simulink model "usrp_4t12r_heatmap"  (R2018a)
settings: Solver=VariableStepDiscrete  StartTime=0.0  StopTime=inf  RelTol=1e-3
undefined symbols (not defined in the file): fft2, gather, get, gpuArray, parula, psBcoor, psWcen, rfcaptureC2Fsim, Time, tsRamp, us
libraries: neural x14, visionanalysis x8, dspobslib x8, dspfdesign x7, dspstat3 x5, dspbuff3 x2, visionsinks x2, commsdrhw_v2 x1, visiontextngfix x1, dspvision x1, visiontransforms x1, dspsigops x1
(part 1 of 4)
settings Model: SimulationMode=accelerator  Creator=Sky  LastModifiedBy=Sky
settings DataIOCC: SaveTime=off
settings OptimizationCC: DefaultUnderspecifiedDataType=single  EfficientMapNaN2IntZero=off  SimCompilerOptimization=on
settings DebuggingCC: ReadBeforeWriteMsg=DisableAll  WriteAfterWriteMsg=DisableAll  WriteAfterReadMsg=DisableAll  MultiTaskDSMMsg=none
settings HardwareCC: TargetBitPerPointer=64  TargetBitPerSizeT=64  TargetBitPerPtrDiffT=64  TargetLongLongMode=on  TargetIntDivRoundTo=Zero  TargetEndianess=LittleEndian  TargetWordSize=64  TargetHWDeviceType=MATLAB Host  ProdEqTarget=off
settings ModelReferenceCC: UpdateModelReferenceTargets=IfOutOfDate
settings SFSimCC: SFSimEcho=off
settings CodeAppCC: MaxIdLength=128  StateflowObjectComments=on
settings GRTTargetCC: TargetLangStandard=C89/C90 (ANSI)  CombineOutputUpdateFcns=off  GRTInterface=on

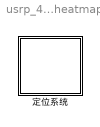
== system usrp_4t12r_heatmap ==
  定位系统 : Subsystem  mask{doSaveParam=on, mode=imaging mode, decimInterp=100, rxBits=logical(dec2bin(0:11)-48), txBits=logical(dec2bin(0:3)-48), rxCoor=single([linspace(-0.053*(12/2-0.5),0.053*(12/2-0.5),12)',zeros(12,2)]), txCoor=single([zeros(4,2),linspace(-0.138-0.053*3,-0.138,4)']), dCa=4.65+0.5, fRamp=2000, fCen=3.2e9, fBw=1e9, tPul=0.025e-3, trEdge=0, trThres=0, yLoDownFac=5, nCyclePF=4, lFftAng=64, lFftDis=128, tDelay=0.5, sFileBack='..\data\yLoCut_4t12r_background.mat', xMi=-3, xMa=3, yMi=1, yMa=4, zMi=-1.25, zMa=0.25, dxC=0.25, dyC=0.25, dzC=0.25, C2Fw=3, C2Fn=2, C2Fratio=0.5, lxW=1, lyW=1, lzW=1.5, tSam=3, nSam=3}
      mask prompts: doSaveParam "save parameters to workspace"; decimInterp "decimation factor"; rxBits "Rx bits"; txBits "Tx bits"; rxCoor "rx coordinates"; txCoor "tx coordinates"; dCa "cable length"; fRamp "ramp frequency"; fCen "center frequency"; fBw "bandwidth"; tPul "pulse width"; trEdge "triger edge"; trThres "triger threshold"; yLoDownFac "yLo downsample factor"; nCyclePF "cycles per frame (average time)"; lFftAng "angle FFT length"; lFftDis "dis FFT length"; tDelay "delay time"; sFileBack "background file path"; xMi "x min"; xMa "x max"; yMi "y min"; yMa "y max"; zMi "z min"; zMa "z max"; dxC "delta x coarse"; dyC "delta y coarse"; dzC "delta z coarse"; C2Fw "coarse to fine width"; C2Fn "coarse to fine cycle number"; C2Fratio "coarse to fine ratio"; lxW "window width x"; lyW "window width y"; lzW "window width z"; tSam "sample time"; nSam "sample number"
      mask init:
      | % Use get_param to obtain the selected string
      | mode = get_param(gcb,'mode');
      | 
      | if strcmp(mode,'get background mode') ...
      |         || strcmp(mode,'sample mode')
      |     evalin('base','clear');
      | end
      | 
      | % 天线和斜坡参数
      | nRx=size(rxBits,1);
      | nTx=size(txBits,1);
      | lFraw=100e6/decimInterp/fRamp*nRx*nTx*nCyclePF;
      | fSraw=100e6/decimInterp;
      | fSdown=fSraw/yLoDownFac;
      | fF=fSraw/lFraw;
      | lRampRaw=fSraw/fRamp;%length ramp raw
      | lRampDown=lRampRaw/yLoDownFac;%length ramp downsample
      | nPul=size(rxBits,2)+size(txBits,2)+1;
      | lPul=fSraw*tPul;%length pulse
      | 
      | dLambda=3e8/fCen;
      | fPm=fBw*fRamp/3e8;%frequency per meter
      | fD=fSdown/lFftDis;%frequency delta
      | fs=single(linspace(0,fSraw/yLoDownFac/2-fD,floor(lFftDis/2)));
      | ds=fs/fPm;
      | 
      | angMax=asind(dLambda/2/abs(rxCoor(1,1)-rxCoor(2,1)));
      | angs=single(linspace(-angMax,angMax,lFftAng));
      | 
      | % 排除线缆长度，截取有效距离
      | dsVal=(ds(ds>=dCa)-dCa)/2;
      | isDval=single(find(dsVal>=yMi & dsVal<=sqrt(yMa^2+((xMa-xMi)/2)^2)));
      | dsVal=dsVal(isDval);
      | isDval=isDval+find(ds>=dCa,1)-1;
      | 
      | % 一个斜坡内的时间
      | tsRampDown=single((0:lRampRaw/yLoDownFac-1)/fSraw*yLoDownFac);
      | isDown=yLoDownFac:yLoDownFac:lFraw;
      | 
      | % 由粗到细成像算法
      | % 读取背景。如果在背景建模模式，设置背景为空白
      | if strcmp(mode,'get background mode')
      |     preciFac=C2Fw.^(C2Fn-1);
      |     xsB=single(xMi:dxC/preciFac:xMa);
      |     ysB=single(yMi:dyC/preciFac:yMa);
      |     zsB=single(zMi:dzC/preciFac:zMa);
      |     [xssB,yssB,zssB]=meshgrid(xsB,ysB,zsB);
      |     
      |     psB=zeros(size(xssB),'single');
      | elseif strcmp(mode,'imaging mode') ...
      |         || strcmp(mode,'sample mode')
      |     load(sFileBack, ...
      |         'xsB','ysB','zsB','xssB','yssB','zssB','psB');
      | end
      | 
      | % 延时样本点数计算
      | lDelay=round(tDelay*fF);
      | 
      | % 分类样本点数计算
      | lSam=length(-round(tSam*fF/2):round(tSam*fF/2));
      | 
      | % 准备窗口坐标
      | psWl=single([lxW,lyW,lzW]);
      | psWdC=single([dxC,dyC,dzC]);
      | 
      | preciFac=C2Fw^(C2Fn-1);
      | dxF=psWdC(1)/preciFac;
      | dyF=psWdC(2)/preciFac;
      | dzF=psWdC(3)/preciFac;
      | xsF=single(-psWl(1)/2:dxF:psWl(1)/2);
      | ysF=single(-psWl(2)/2:dyF:psWl(2)/2);
      | zsF=single(-psWl(3)/2:dzF:psWl(3)/2);
      | sizePsF=[length(ysF),length(xsF),length(zsF)];
      | 
      | % 保存参数到工作空间base
      | if doSaveParam
      |     % mask变量
      |     assignin('base','rxBits',rxBits);
      |     assignin('base','txBits',txBits);
      |     assignin('base','rxCoor',rxCoor);
      |     assignin('base','txCoor',txCoor);
      |     assignin('base','dCa',dCa);
      |     assignin('base','fRamp',fRamp);
      |     assignin('base','fCen',fCen);
      |     assignin('base','fBw',fBw);
      |     assignin('base','tPul',tPul);
      |     assignin('base','yLoDownFac',yLoDownFac);
      |     assignin('base','nCyclePF',nCyclePF);
      |     assignin('base','lFftAng',lFftAng);
      |     assignin('base','lFftDis',lFftDis);
      |     assignin('base','tDelay',tDelay);
      |     assignin('base','sFileBack',sFileBack);
      |     
      |     assignin('base','mode',mode);
      |     assignin('base','xMi',xMi);
      |     assignin('base','xMa',xMa);
      |     assignin('base','yMi',yMi);
      |     assignin('base','yMa',yMa);
      |     assignin('base','zMi',zMi);
      |     assignin('base','zMa',zMa);
      |     assignin('base','dxC',dxC);
      |     assignin('base','dyC',dyC);
      |     assignin('base','dzC',dzC);
      |     assignin('base','C2Fw',C2Fw);
      |     assignin('base','C2Fn',C2Fn);
      |     assignin('base','C2Fratio',C2Fratio);
      |     assignin('base','tSam',tSam);
      |     assignin('base','nSam',nSam);
      |     
      |     % 全局变量
      |     assignin('base','nRx',nRx);
      |     assignin('base','nTx',nTx);
      |     assignin('base','lFraw',lFraw);
      |     assignin('base','fF',fF);
      |     assignin('base','fSraw',fSraw);
      |     assignin('base','fSdown',fSdown);
      |     assignin('base','fPm',fPm);
      |     assignin('base','lRampRaw',lRampRaw);
      |     assignin('base','dLambda',dLambda);
      |     assignin('base','ds',ds);
      |     assignin('base','angs',angs);
      |     assignin('base','dsVal',dsVal);
      |     assignin('base','isDval',isDval);
      |     assignin('base','tsRamp',tsRampDown);
      |     assignin('base','dxF',dxF);
      |     assignin('base','dyF',dyF);
      |     assignin('base','dzF',dzF);
      |     assignin('base','xsF',xsF);
      |     assignin('base','ysF',ysF);
      |     assignin('base','zsF',zsF);
      |     assignin('base','psWl',psWl);
      |     assignin('base','psWdC',psWdC);
      |     assignin('base','lDelay',lDelay);
      |     assignin('base','lSam',lSam);
      | end
      mask TypeOptions mode: get background mode | imaging mode | sample mode
      mask TypeOptions decimInterp: USRP/decimInterp
      mask DialogControl simParam Prompt: sim parameters
      mask DialogControl USRPparams Prompt: USRP Parameters
      mask DialogControl hwParams Prompt: Hardware Parameters
      mask DialogControl rampParams Prompt: Ramp Parameters
      mask DialogControl preParams Prompt: Preprocess Parameters
      mask DialogControl fftParams Prompt: FFT Parameters
      mask DialogControl imagParams Prompt: Imaging Parameters
      mask DialogControl samParams Prompt: Sample Parameters
      mask Display: disp('定位系统');

== system usrp_4t12r_heatmap/定位系统 ==
  USRP : Subsystem  mask{decimInterp=decimInterp, lF=lFraw}
      mask prompts: decimInterp "Decimation Factor"; lF "frameLength"
      mask TypeOptions decimInterp: SDRu Receiver/decimInterp
      mask TypeOptions lF: SDRu Receiver/frameLength
      mask Display: disp('USRP');
  定位模块 : Subsystem
  wires:
  USRP/1(Data) -> 定位模块/1(frame)
  USRP/2(Data Len) -> 定位模块/Enable

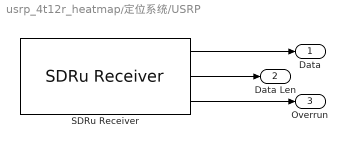
== system usrp_4t12r_heatmap/定位系统/USRP ==
  SDRu Receiver : commsdrhw_v2/SDRu Receiver  SourceLibraryInfo="This block requires <a href=\"http://www.mathworks.com/hardware-support/usrp.html\">Communications System Toolbox Support Package for USRP Radio</a>"  rxtx=rx  initializeIPAddress=0  devMap=0  USRP2_IP=192.168.10.6  USRP_IP_X300=192.168.10.2  USRP_IP_X310=192.168.10.2  USRP_serialNumB200=No devices found  USRP_serialNumB210=No devices found  platform=N200/N210/USRP2  prevPlatform=N200/N210/USRP2  lastIPAddressPopup=192.168.10.2  USRP_ID=192.168.10.6  LastIPAddress=192.168.10.2  ChannelMapping=1  centerFrequencySrc=Dialog  centerFrequency=0  loOffsetSrc=Dialog  loOffset=0  gainSrc=Dialog  gain=0  PPSSource=Internal  clockSource=Internal  masterClkRateParam=100e6  masterClkRateB200=32e6  masterClkRateB210=32e6  masterClkRateX300=200e6  masterClkRateX310=200e6  masterClkRate=100e6  decimInterpSrc=Dialog  decimInterp=decimInterp  USRP2_IP_NUM=[49 57 50 46 49 54 56 46 49 48 46 54]  TransportDataType=int16  overrunUnderrunPort=on  sampleTime=decimInterp/100e6  outputDatatype=single  frameLength=lF  HOST_DATA_PORT=0  HOST_CONTROL_PORT=0  USRP2_DATA_PORT=0  USRP2_CONTROL_PORT=0  bufferMode=Continuous streaming  EnableBurstMode=off  NumFramesInBurst=10000
      settings: SourceProductName=Communications System Toolbox Support Package for USRP(R) Radio  SourceProductBaseCode=USRP
  Data : Outport
  Data Len : Outport  Port=2
  Overrun : Outport  Port=3
  wires:
  SDRu Receiver/2 -> Data Len/1
  SDRu Receiver/3 -> Overrun/1
  SDRu Receiver/1 -> Data/1

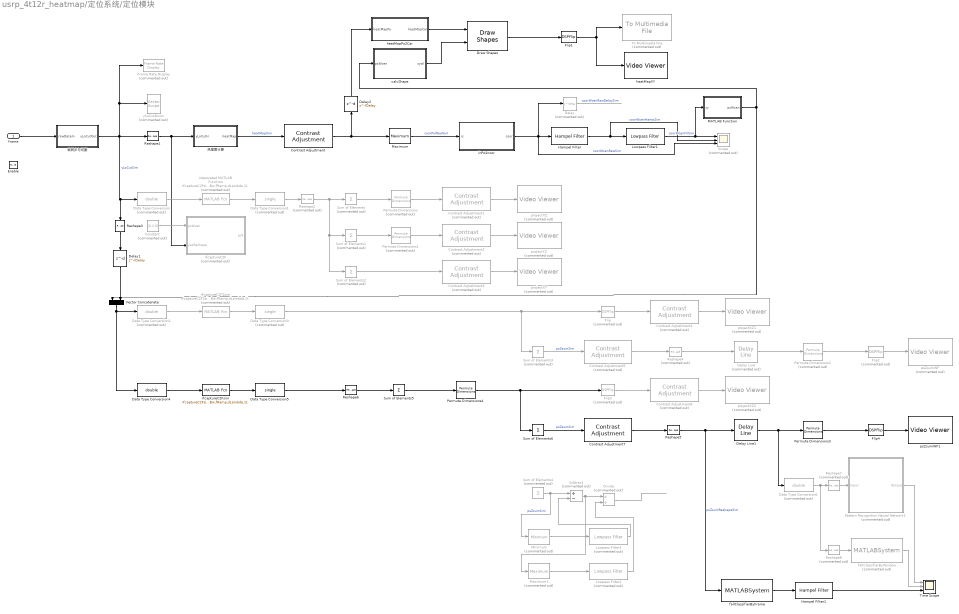
== system usrp_4t12r_heatmap/定位系统/定位模块 ==
  frame : Inport
  Enable : EnablePort  PropagateVarSize=During execution
  Constant : Constant  Commented=on  Value=[0,2,0]  OutDataTypeStr=single
  Contrast Adjustment : visionanalysis/Contrast Adjustment  methodInputRange=Full input data range [min max]  rangeIn=[0 255]  fracSaturate=[1 1]  isBinNum=on  binNum=256  methodOutputRange=Full data type range  rangeOut=[0 255]  prod1Mode=Binary point scaling  prod1WordLength=32  prod1FracLength=16  prod2Mode=Binary point scaling  prod2WordLength=32  prod2FracLength=16  roundingMode=Floor  overflowMode=off
      settings: SourceProductName=Computer Vision System Toolbox  SourceProductBaseCode=VP
  Contrast Adjustment{1..6} (6 alike) : visionanalysis/Contrast Adjustment  Commented=on  methodInputRange=Full input data range [min max]  rangeIn=[0 255]  fracSaturate=[1 1]  isBinNum=on  binNum=256  methodOutputRange=Full data type range  rangeOut=[0 255]  prod1Mode=Binary point scaling  prod1WordLength=32  prod1FracLength=16  prod2Mode=Binary point scaling  prod2WordLength=32  prod2FracLength=16  roundingMode=Floor  overflowMode=off
      settings: SourceProductName=Computer Vision System Toolbox  SourceProductBaseCode=VP
  Contrast Adjustment7 : visionanalysis/Contrast Adjustment  methodInputRange=Full input data range [min max]  rangeIn=[0 255]  fracSaturate=[1 1]  isBinNum=on  binNum=256  methodOutputRange=Full data type range  rangeOut=[0 255]  prod1Mode=Binary point scaling  prod1WordLength=32  prod1FracLength=16  prod2Mode=Binary point scaling  prod2WordLength=32  prod2FracLength=16  roundingMode=Floor  overflowMode=off
      settings: SourceProductName=Computer Vision System Toolbox  SourceProductBaseCode=VP
  Data Type Conversion : DataTypeConversion  Commented=on  OutDataTypeStr=double
  Data Type Conversion1 : DataTypeConversion  Commented=on  OutDataTypeStr=single
  Data Type Conversion2 : DataTypeConversion  Commented=on  OutDataTypeStr=double
  Data Type Conversion3 : DataTypeConversion  Commented=on  OutDataTypeStr=single
  Data Type Conversion4 : DataTypeConversion  OutDataTypeStr=double
  Data Type Conversion5 : DataTypeConversion  OutDataTypeStr=single
  Data Type Conversion6 : DataTypeConversion  Commented=on  OutDataTypeStr=double
  Delay : Delay  Commented=on  DelayLength=lDelay  InitialCondition=0
  Delay Line : dspbuff3/Delay Line  Commented=on  siz=lSam  ic=0  directfeed=off  enable_output=off  hold_output=off  OutputFrames=off
      settings: SourceProductName=DSP System Toolbox  SourceProductBaseCode=DS
  Delay Line1 : dspbuff3/Delay Line  siz=lSam  ic=0  directfeed=off  enable_output=off  hold_output=off  OutputFrames=off
      settings: SourceProductName=DSP System Toolbox  SourceProductBaseCode=DS
  Delay1 : Delay  DelayLength=lDelay  InitialCondition=0
  Delay2 : Delay  DelayLength=lDelay  InitialCondition=0
  Divide : Product  Commented=on  Inputs=*/
  Draw Shapes : visiontextngfix/Draw Shapes  shape=Rectangles  fill=off  lineWidth=1  fillClrSource=Specify via dialog  display=White  intensity=200  color=[200 255 100]  opacity=0.6  viewport=Entire image  antialiasing=off  inType=Obsolete  imagePorts=One multidimensional signal  prodOutputMode=Binary point scaling  prodOutputWordLength=32  prodOutputFracLength=14  memoryMode=Specify word length  memoryWordLength=16  memoryFracLength=15  roundingMode=Floor  overflowMode=off
      settings: SourceProductName=Computer Vision System Toolbox
  Flip : DSPFlip  Commented=on
  Flip1 : DSPFlip  dim=Rows
  Flip2 : DSPFlip  Commented=on
  Flip3 : DSPFlip  Commented=on
  Flip4 : DSPFlip
  Frame Rate Display : visionsinks/Frame Rate Display  Commented=on  UpdateRate=10
      settings: SourceProductName=Computer Vision System Toolbox  SourceProductBaseCode=VP
  Hampel Filter : dspfdesign/Hampel Filter  WindowLength=round(fF/2)*2+1  ThresholdPort=off  Threshold=0.2  EnableIsOutlierOutput=off  SimulateUsing=Code generation
      settings: SourceProductName=DSP System Toolbox  SourceProductBaseCode=DS
  Hampel Filter1 : dspfdesign/Hampel Filter  WindowLength=round(fF/2)*2+1  ThresholdPort=off  Threshold=0.2  EnableIsOutlierOutput=off  SimulateUsing=Code generation
      settings: SourceProductName=DSP System Toolbox  SourceProductBaseCode=DS
  Interpreted MATLAB Function : MATLABFcn  Commented=on  MATLABFcn=rfcaptureC2Fsim(psWcen,psWl,psWdC,psBcoor,psB,C2Fratio,C2Fw,C2Fn,single(u),rxCoor,txCoor,nRx,tsRampDown,fBw,fRamp,dLambda,1);  OutputSignalType=real  Output1D=off
  Lowpass Filter1 : dspfdesign/Lowpass Filter  FilterType=IIR  DesignForMinimumOrder=off  FilterOrder=1  PassbandFrequency=0.5  StopbandFrequency=3  PassbandRipple=0.1  StopbandAttenuation=30  InheritSampleRate=off  SampleRate=fF  SimulateUsing=Code generation  roundingMode=Floor  coeffsDataTypeStr=fixdt(1,16)
  Lowpass Filter2 : dspfdesign/Lowpass Filter  Commented=on  FilterType=IIR  DesignForMinimumOrder=off  FilterOrder=1  PassbandFrequency=0.5  StopbandFrequency=3  PassbandRipple=0.1  StopbandAttenuation=30  InheritSampleRate=off  SampleRate=fF  SimulateUsing=Interpreted execution  roundingMode=Floor  coeffsDataTypeStr=fixdt(1,16)
  Lowpass Filter3 : dspfdesign/Lowpass Filter  Commented=on  FilterType=IIR  DesignForMinimumOrder=off  FilterOrder=1  PassbandFrequency=0.5  StopbandFrequency=3  PassbandRipple=0.1  StopbandAttenuation=30  InheritSampleRate=off  SampleRate=fF  SimulateUsing=Interpreted execution  roundingMode=Floor  coeffsDataTypeStr=fixdt(1,16)
  MATLAB Function : MATLAB Function  TreatAsAtomicUnit=on
  Maximum : dspstat3/Maximum  operation=maximum  fcn=Index  indexBase=One  operateOver=Entire input  Dimension=1  InputProcessing=Columns as channels (frame based)  reset=None  roiEnable=off  roiType=Rectangles  roiPortion=Entire ROI  roiOutput=Individual statistics for each ROI  roiFlag=off  roundingMode=Floor  overflowMode=off  accumDataTypeStr=Inherit: Same as product output  accumLastDataTypeStr=Inherit: Same as product output
  Maximum1 : dspstat3/Maximum  Commented=on  operation=maximum  fcn=Value  indexBase=One  operateOver=Entire input  Dimension=1  InputProcessing=Columns as channels (frame based)  reset=None  roiEnable=off  roiType=Rectangles  roiPortion=Entire ROI  roiOutput=Individual statistics for each ROI  roiFlag=off  roundingMode=Floor  overflowMode=off  accumDataTypeStr=Inherit: Same as product output  accumLastDataTypeStr=Inherit: Same as product output
  Minimum : dspstat3/Minimum  Commented=on  operation=minimum  fcn=Value  indexBase=One  operateOver=Entire input  Dimension=1  InputProcessing=Columns as channels (frame based)  reset=None  roiEnable=off  roiType=Rectangles  roiPortion=Entire ROI  roiOutput=Individual statistics for each ROI  roiFlag=off  roundingMode=Floor  overflowMode=off
      settings: SourceProductName=DSP System Toolbox  SourceProductBaseCode=DS
  Pattern Recognition Neural Network1 : Subsystem  Commented=on
      mask help: Pattern Recognition Neural Network
      mask Display: e = 0.06;c1 = [120 150 230]/255;c2 = ([120 150 230]+0)/383;c3 = ([120 150 230]+128)/383;patch([0 1 1 0],[0 0 1 1],c1);patch([0 1 1 1-e 1-e 0+e],[0 0 1 1-e 0+e 0+e],c2);patch([0 0 1 1-e 0+e 0+e],[0 1 1 1-e 1-e 0+e],c3);plot([0 1 1 0 0],[0 0 1 1 0]);fprintf('NNET');port_label('input',1,' Input');port_label('output',1,'Output ');
  Permute Dimensions : PermuteDimensions  Commented=on  Order=[3,2,1]
  Permute Dimensions1 : PermuteDimensions  Commented=on  Order=[3,1,2]
  Permute Dimensions2 : PermuteDimensions  Commented=on
  Permute Dimensions3 : PermuteDimensions
  Permute Dimensions4 : PermuteDimensions  Order=[3,2,1]
  Reshape1 : Reshape  OutputDimensionality=Customize  OutputDimensions=[lRampDown,nRx,nTx]
  Reshape2 : Reshape  Commented=on  OutputDimensionality=Customize  OutputDimensions=[length(ysF),length(xsF),length(zsF)]
  Reshape3 : Reshape  OutputDimensionality=Row vector (2-D)  OutputDimensions=[lRampDown,nRx,nTx]
  Reshape4 : Reshape  Commented=on  OutputDimensionality=Row vector (2-D)  OutputDimensions=[lRampDown,nRx,nTx]
  Reshape5 : Reshape  OutputDimensionality=Row vector (2-D)  OutputDimensions=[lRampDown,nRx,nTx]
  Reshape6 : Reshape  OutputDimensionality=Customize  OutputDimensions=[length(ysF),length(xsF),length(zsF)]
  Reshape7 : Reshape  Commented=on  OutputDimensionality=Column vector (2-D)  OutputDimensions=[lRampDown,nRx,nTx]
  Reshape8 : Reshape  Commented=on  OutputDimensionality=Row vector (2-D)  OutputDimensions=[lRampDown,nRx,nTx]
  Scope : Scope  Commented=on  NumInputPorts=3
  Subtract : Sum  Commented=on  Inputs=+-
  Sum of Elements : Sum  Commented=on  Inputs=+  CollapseMode=Specified dimension
  Sum of Elements1 : Sum  Commented=on  Inputs=+  CollapseMode=Specified dimension  CollapseDim=2
  Sum of Elements2 : Sum  Commented=on  Inputs=+  CollapseMode=Specified dimension  CollapseDim=3
  Sum of Elements3 : Sum  Commented=on  Inputs=+  CollapseMode=Specified dimension  CollapseDim=2
  Sum of Elements4 : Sum  Commented=on  Inputs=+  CollapseMode=Specified dimension  CollapseDim=2
  Sum of Elements5 : Sum  Inputs=+  CollapseMode=Specified dimension
  Sum of Elements6 : Sum  Inputs=+  CollapseMode=Specified dimension  CollapseDim=2
  Time Scope : Scope  NumInputPorts=3
  To Multimedia File : dspvision/To Multimedia File  Commented=on  outputFilename=..\..\heatMap.avi  streamSelection=Video only  videoCompressor=MJPEG Compressor  audioCompressor=None (uncompressed)  imagePorts=One multidimensional signal  fileType=AVI  audioDatatype=Determine from input data type  fourcc=RGB  videoQuality=85  mj2000CompFactor=10
      settings: SourceProductName=Computer Vision System Toolbox  SourceProductBaseCode=VP
  Vector Concatenate : Concatenate
  calcShape : MATLAB Function  TreatAsAtomicUnit=on
  fallClassifierByFrame : MATLABSystem  System=fallClassifierByFrame  SimulateUsing=Code generation
      mask Type: fallClassifierByFrame
      mask Display:
      | disp('fallClassifierByFrame');
      | port_label('input',1,'u');
      | port_label('output',1,'y');
  fallClassifierByWindow : MATLABSystem  Commented=on  System=fallClassifierByWindow  SimulateUsing=Code generation
      mask Type: fallClassifierByWindow
      mask Display:
      | disp('fallClassifierByWindow');
      | port_label('input',1,'u');
      | port_label('output',1,'y');
  heatMapPo2Car : MATLAB Function  TreatAsAtomicUnit=on
  heatMapXY : VideoViewer  useColorMap=on  colormapValue=parula(256)  FigPos=[962 1037 958 408]
  inPo2coor : MATLAB Function  TreatAsAtomicUnit=on
  projectXY : VideoViewer  Commented=on  useColorMap=on  colormapValue=parula(256)  FigPos=[2 517 958 408]
  projectXZ : VideoViewer  Commented=on  useColorMap=on  colormapValue=parula(256)  FigPos=[2 1037 958 408]
  projectXZ1 : VideoViewer  Commented=on  useColorMap=on  colormapValue=parula(256)  FigPos=[962 517 958 408]
  projectXZ2 : VideoViewer  Commented=on  useColorMap=on  colormapValue=parula(256)  FigPos=[2 517 958 408]
  projectYZ : VideoViewer  Commented=on  useColorMap=on  colormapValue=parula(256)  FigPos=[962 517 958 408]
  psZsumWF : VideoViewer  Commented=on  useColorMap=on  colormapValue=parula(256)  FigPos=[2 517 958 408]
  psZsumWF1 : VideoViewer  useColorMap=on  colormapValue=parula(256)  FigPos=[962 517 958 408]
  rfcaptureC2F : MATLAB Function  Commented=on  TreatAsAtomicUnit=on
  rfcaptureC2F2sim : MATLABFcn  Commented=on  MATLABFcn=rfcaptureC2F2sim(single(u(1:3)),psWl,psWdC,xssB,yssB,zssB,psB,C2Fratio,C2Fw,C2Fn,single(u(4:end)),rxCoor,txCoor,dCa,tsRampDown,fBw,fRamp,dLambda,1);  OutputDimensions=[length(zsF),length(xsF)]  Output1D=off
  rfcaptureC2Fsim : MATLABFcn  MATLABFcn=rfcaptureC2Fsim(single(u(1:3)),psWl,psWdC,xssB,yssB,zssB,psB,C2Fratio,C2Fw,C2Fn,single(u(4:end)),rxCoor,txCoor,dCa,tsRampDown,fBw,fRamp,dLambda,1);  OutputDimensions=[length(xsF)*length(ysF)*length(zsF),1]  Output1D=off
  yLoCutDown : dspobslib/Vector Scope  Commented=on  ScopeProperties=on  Domain=User-defined  HorizSpan=1  DisplayProperties=off  AxisGrid=on  Memory=off  FrameNumber=on  AxisLegend=off  AxisZoom=off  OpenScopeAtSimStart=on  OpenScopeImmediately=off  FigPos=get(0,'defaultfigureposition')  AxisProperties=off  XUnits=Hertz  XRange=[0...Fs/2]  InheritXIncr=off  XIncr=1e6/fSdown  XLabel=Time(us)  XLimit=Auto  XMin=0  XMax=1  XStart=0  YUnits=dB  YLabel=Amplitude  LineProperties=off  LineColors=[1 0 0]|[0 1 0]|[0 0 1]  XAxisParamsVer=6.9
      settings: SourceProductName=DSP System Toolbox  SourceProductBaseCode=DS  YMin=-0.3  YMax=0.3
  帧同步与切割 : Subsystem
  热度图计算 : Subsystem
  wires:
  frame/1 -> 帧同步与切割/1(rawDateIn)
  热度图计算/1(heatMap) -> Contrast Adjustment/1  "heatMapSim"
  Maximum/1 -> inPo2coor/1(is)  "coorPolRawSim"
  Lowpass Filter1/1 -> MATLAB Function/1(xy), Scope/1  "coorWcenFilSim"
  Hampel Filter/1 -> Scope/2, Lowpass Filter1/1  "coorWcenHampSim"
  Contrast Adjustment/1 -> Maximum/1, Delay2/1
  inPo2coor/1(coor) -> Delay/1, Scope/3, Hampel Filter/1  "coorWcenRawSim"
  Reshape1/1 -> rfcaptureC2F/2(yLoReshape), 热度图计算/1(yLoCutIn)
  Constant/1 -> rfcaptureC2F/1(psWcen)
  Interpreted MATLAB Function/1 -> Data Type Conversion1/1
  Sum of Elements/1 -> Permute Dimensions/1
  Permute Dimensions/1 -> Contrast Adjustment1/1
  Data Type Conversion/1 -> Interpreted MATLAB Function/1
  Contrast Adjustment1/1 -> projectXZ/1
  Sum of Elements1/1 -> Permute Dimensions1/1
  Permute Dimensions1/1 -> Contrast Adjustment2/1
  Contrast Adjustment2/1 -> projectYZ/1
  Reshape2/1 -> Sum of Elements2/1, Sum of Elements1/1, Sum of Elements/1
  Contrast Adjustment3/1 -> projectXY/1
  Sum of Elements2/1 -> Contrast Adjustment3/1
  Data Type Conversion1/1 -> Reshape2/1
  帧同步与切割/1(yLoCutOut) -> Data Type Conversion/1, Reshape3/1, Reshape1/1, Frame Rate Display/1, yLoCutDown/1  "yLoCutSim"
  Data Type Conversion3/1 -> Flip/1, Sum of Elements3/1
  Contrast Adjustment4/1 -> projectXZ1/1
  Data Type Conversion2/1 -> rfcaptureC2F2sim/1
  rfcaptureC2F2sim/1 -> Data Type Conversion3/1
  Sum of Elements3/1 -> Contrast Adjustment5/1  "psZsumSim"
  Flip/1 -> Contrast Adjustment4/1
  Delay/1 -> ?  "coorWcenRawDelaySim"
  Delay Line/1 -> Permute Dimensions2/1
  Vector Concatenate/1 -> Data Type Conversion4/1, Data Type Conversion2/1
  Reshape3/1 -> Delay1/1
  Delay1/1 -> Vector Concatenate/2
  heatMapPo2Car/1(heatMapCar) -> Draw Shapes/1
  Delay2/1 -> heatMapPo2Car/1(heatMapPo)
  MATLAB Function/1(psWcen) -> calcShape/1(psWcen), Vector Concatenate/1
  Flip1/1 -> To Multimedia File/1, heatMapXY/1
  Draw Shapes/1 -> Flip1/1
  calcShape/1(xywl) -> Draw Shapes/2
  Contrast Adjustment5/1 -> Reshape4/1
  Permute Dimensions2/1 -> Flip2/1
  Flip2/1 -> psZsumWF/1
  Reshape4/1 -> Delay Line/1
  Permute Dimensions3/1 -> Flip4/1
  Delay Line1/1 -> Data Type Conversion6/1, Permute Dimensions3/1
  Flip4/1 -> psZsumWF1/1
  Reshape5/1 -> fallClassifierByFrame/1, Delay Line1/1  "psZsumReshapeSim"
  rfcaptureC2Fsim/1 -> Data Type Conversion5/1
  Flip3/1 -> Contrast Adjustment6/1
  Data Type Conversion4/1 -> rfcaptureC2Fsim/1
  Data Type Conversion5/1 -> Reshape6/1
  Contrast Adjustment6/1 -> projectXZ2/1
  Reshape6/1 -> Sum of Elements5/1
  Sum of Elements5/1 -> Permute Dimensions4/1
  Contrast Adjustment7/1 -> Reshape5/1
  Sum of Elements6/1 -> Contrast Adjustment7/1  "psZsumSim"
  Permute Dimensions4/1 -> Sum of Elements6/1, Flip3/1
  Divide/1 -> ?
  Maximum1/1 -> Lowpass Filter2/1
  Lowpass Filter2/1 -> Divide/2
  Subtract/1 -> Divide/1, Maximum1/1
  ? -> Sum of Elements4/1
  Lowpass Filter3/1 -> Subtract/2
  Minimum/1 -> Lowpass Filter3/1
  Sum of Elements4/1 -> Minimum/1, Subtract/1  "psZsumSim"
  fallClassifierByFrame/1 -> Hampel Filter1/1
  Hampel Filter1/1 -> Time Scope/3
  Pattern Recognition Neural Network1/1(Output) -> Time Scope/1
  Data Type Conversion6/1 -> Reshape7/1, Reshape8/1
  fallClassifierByWindow/1 -> Time Scope/2
  Reshape7/1 -> Pattern Recognition Neural Network1/1(Input)
  Reshape8/1 -> fallClassifierByWindow/1

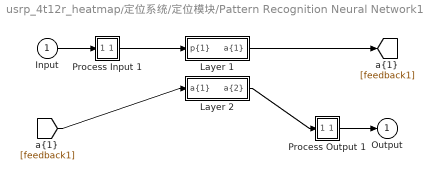
== system usrp_4t12r_heatmap/定位系统/定位模块/Pattern Recognition Neural Network1 ==
  Input : Inport  PortDimensions=627
      mask Display: e = 0.06;c1 = [120 230 180]/255;c2 = ([120 230 180]+0)/(256+128);c3 = ([120 230 180]+128)/(256+128);patch([0 1 1 0],[0 0 1 1],c1);patch([0 1 1 1-e 1-e 0+e],[0 0 1 1-e 0+e 0+e],c2);patch([0 0 1 1-e 0+e 0+e],[0 1 1 1-e 1-e 0+e],c3);plot([0 1 1 0 0],[0 0 1 1 0]);
  Layer 1 : Subsystem
      mask Display: e = 0.06;c1 = [120 150 230]/255;c2 = ([120 150 230]+0)/383;c3 = ([120 150 230]+128)/383;patch([0 1 1 0],[0 0 1 1],c1);patch([0 1 1 1-e 1-e 0+e],[0 0 1 1-e 0+e 0+e],c2);patch([0 0 1 1-e 0+e 0+e],[0 1 1 1-e 1-e 0+e],c3);plot([0 1 1 0 0],[0 0 1 1 0]);
  Layer 2 : Subsystem
      mask Display: e = 0.06;c1 = [120 150 230]/255;c2 = ([120 150 230]+0)/383;c3 = ([120 150 230]+128)/383;patch([0 1 1 0],[0 0 1 1],c1);patch([0 1 1 1-e 1-e 0+e],[0 0 1 1-e 0+e 0+e],c2);patch([0 0 1 1-e 0+e 0+e],[0 1 1 1-e 1-e 0+e],c3);plot([0 1 1 0 0],[0 0 1 1 0]);
  Process Input 1 : Subsystem
      mask Display: e = 0.06;c1 = [120 150 230]/255;c2 = ([120 150 230]+0)/383;c3 = ([120 150 230]+128)/383;patch([0 1 1 0],[0 0 1 1],c1);patch([0 1 1 1-e 1-e 0+e],[0 0 1 1-e 0+e 0+e],c2);patch([0 0 1 1-e 0+e 0+e],[0 1 1 1-e 1-e 0+e],c3);plot([0 1 1 0 0],[0 0 1 1 0]);
  Process Output 1 : Subsystem
      mask Display: e = 0.06;c1 = [120 150 230]/255;c2 = ([120 150 230]+0)/383;c3 = ([120 150 230]+128)/383;patch([0 1 1 0],[0 0 1 1],c1);patch([0 1 1 1-e 1-e 0+e],[0 0 1 1-e 0+e 0+e],c2);patch([0 0 1 1-e 0+e 0+e],[0 1 1 1-e 1-e 0+e],c3);plot([0 1 1 0 0],[0 0 1 1 0]);
  Output : Outport  InitialOutput=0
      mask Display: e = 0.06;c1 = [120 230 180]/255;c2 = ([120 230 180]+0)/(256+128);c3 = ([120 230 180]+128)/(256+128);patch([0 1 1 0],[0 0 1 1],c1);patch([0 1 1 1-e 1-e 0+e],[0 0 1 1-e 0+e 0+e],c2);patch([0 0 1 1-e 0+e 0+e],[0 1 1 1-e 1-e 0+e],c3);plot([0 1 1 0 0],[0 0 1 1 0]);
  wires:
  Input/1 -> Process Input 1/1(x)
  Process Output 1/1(y) -> Output/1
  Process Input 1/1(p) -> Layer 1/1("p{1}")
  Layer 1/1("a{1}") -> [feedback1]
  [feedback1] -> Layer 2/1("a{1} ")
  Layer 2/1("a{2}") -> Process Output 1/1(a)

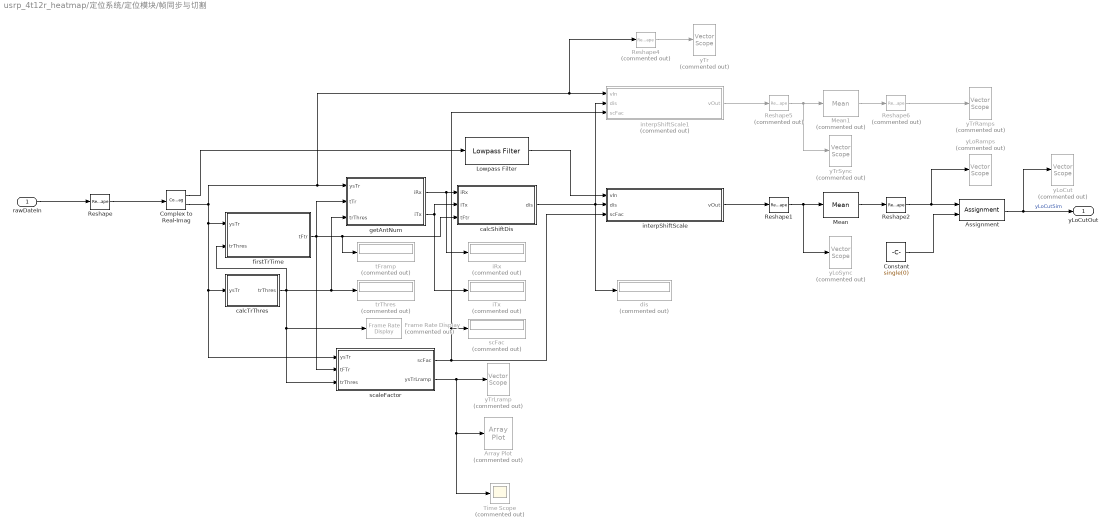
== system usrp_4t12r_heatmap/定位系统/定位模块/帧同步与切割 ==
  rawDateIn : Inport
  Array Plot : ArrayPlot  Commented=on
  Assignment : Assignment  NumberOfDimensions=2  DiagnosticForDimensions=Warning  IndexOptions=Index vector (dialog),Assign all  Indices=[1:ceil(2e-5*fSdown),lRampDown-ceil(2e-5*fSdown):lRampDown],1  OutputSizes=1,1
  Complex to Real-Imag : ComplexToRealImag
  Constant : Constant  Value=single(0)
  Frame Rate Display : visionsinks/Frame Rate Display  Commented=on  UpdateRate=10
      settings: SourceProductName=Computer Vision System Toolbox  SourceProductBaseCode=VP
  Lowpass Filter : dspfdesign/Lowpass Filter  FilterType=FIR  DesignForMinimumOrder=on  FilterOrder=20  PassbandFrequency=0.3*fSdown  StopbandFrequency=min(0.7*fSdown,0.5*fSraw)  PassbandRipple=0.1  StopbandAttenuation=50  InheritSampleRate=off  SampleRate=fSraw  SimulateUsing=Interpreted execution  roundingMode=Floor  coeffsDataTypeStr=fixdt(1,16)
  Mean : dspstat3/Mean  run=off  InputProcessing=Columns as channels (frame based)  reset_popup=None  directionMode=Each row  dimension=1  roiEnable=off  roiType=Rectangles  roiPortion=Entire ROI  roiOutput=Individual statistics for each ROI  roiFlag=off  roundingMode=Floor  overflowMode=off  outputDataTypeStr=Inherit: Same as accumulator  outputMin=[]  outputMax=[]  outputLastDataTypeStr=Inherit: Same as accumulator
  Mean1 : dspstat3/Mean  Commented=on  run=off  InputProcessing=Columns as channels (frame based)  reset_popup=None  directionMode=Each row  dimension=1  roiEnable=off  roiType=Rectangles  roiPortion=Entire ROI  roiOutput=Individual statistics for each ROI  roiFlag=off  roundingMode=Floor  overflowMode=off  outputDataTypeStr=Inherit: Same as accumulator  outputMin=[]  outputMax=[]  outputLastDataTypeStr=Inherit: Same as accumulator
  Reshape : Reshape  OutputDimensionality=Column vector (2-D)
  Reshape1 : Reshape  OutputDimensionality=Customize  OutputDimensions=[lRampDown*nRx*nTx,nCyclePF]
  Reshape2 : Reshape  OutputDimensionality=Customize  OutputDimensions=[lRampDown,nRx*nTx]
  Reshape4 : Reshape  Commented=on  OutputDimensionality=Column vector (2-D)
  Reshape5 : Reshape  Commented=on  OutputDimensionality=Customize  OutputDimensions=[lRampDown*nRx*nTx,nCyclePF]
  Reshape6 : Reshape  Commented=on  OutputDimensionality=Customize  OutputDimensions=[lRampDown,nRx*nTx]
  Time Scope : Scope  Commented=on
  calcShiftDis : MATLAB Function  TreatAsAtomicUnit=on
  calcTrThres : MATLAB Function  TreatAsAtomicUnit=on
  dis : Display  Commented=on
  firstTrTime : MATLAB Function  TreatAsAtomicUnit=on
  getAntNum : MATLAB Function  TreatAsAtomicUnit=on
  iRx : Display  Commented=on
  iTx : Display  Commented=on
  interpShiftScale : MATLAB Function  TreatAsAtomicUnit=on
  interpShiftScale1 : MATLAB Function  Commented=on  TreatAsAtomicUnit=on
  scFac : Display  Commented=on
  scaleFactor : MATLAB Function  TreatAsAtomicUnit=on
  tFramp : Display  Commented=on
  trThres : Display  Commented=on
  yLoCut : dspobslib/Vector Scope  Commented=on  ScopeProperties=on  Domain=User-defined  HorizSpan=1  DisplayProperties=off  AxisGrid=on  Memory=off  FrameNumber=on  AxisLegend=off  AxisZoom=off  OpenScopeAtSimStart=on  OpenScopeImmediately=off  FigPos=get(0,'defaultfigureposition')  AxisProperties=off  XUnits=Hertz  XRange=[0...Fs/2]  InheritXIncr=off  XIncr=1e6/fSdown  XLabel=Time(us)  XLimit=Auto  XMin=0  XMax=1  XStart=0  YUnits=dB  YLabel=Amplitude  LineProperties=off  LineColors=[1 0 0]|[0 1 0]|[0 0 1]  XAxisParamsVer=6.9
      settings: SourceProductName=DSP System Toolbox  SourceProductBaseCode=DS  YMin=-0.3  YMax=0.3
  yLoRamps : dspobslib/Vector Scope  Commented=on  ScopeProperties=on  Domain=User-defined  HorizSpan=1  DisplayProperties=off  AxisGrid=on  Memory=off  FrameNumber=on  AxisLegend=off  AxisZoom=off  OpenScopeAtSimStart=on  OpenScopeImmediately=off  FigPos=get(0,'defaultfigureposition')  AxisProperties=off  XUnits=Hertz  XRange=[0...Fs/2]  InheritXIncr=off  XIncr=1e6/fSdown  XLabel=Time(us)  XLimit=Auto  XMin=0  XMax=1  XStart=0  YUnits=dB  YLabel=Amplitude  LineProperties=off  LineColors=[1 0 0]|[0 1 0]|[0 0 1]  XAxisParamsVer=6.9
      settings: SourceProductName=DSP System Toolbox  SourceProductBaseCode=DS  YMin=-0.3  YMax=0.3
  yLoSync : dspobslib/Vector Scope  Commented=on  ScopeProperties=on  Domain=User-defined  HorizSpan=1  DisplayProperties=off  AxisGrid=on  Memory=off  FrameNumber=on  AxisLegend=off  AxisZoom=off  OpenScopeAtSimStart=on  OpenScopeImmediately=off  FigPos=get(0,'defaultfigureposition')  AxisProperties=off  XUnits=Hertz  XRange=[0...Fs/2]  InheritXIncr=off  XIncr=1e6/fSdown  XLabel=Time(us)  XLimit=Auto  XMin=0  XMax=1  XStart=0  YUnits=dB  YLabel=Amplitude  LineProperties=off  LineColors=[1 0 0]|[0 1 0]|[0 0 1]  XAxisParamsVer=6.9
      settings: SourceProductName=DSP System Toolbox  SourceProductBaseCode=DS  YMin=-0.3  YMax=0.3
  yTr : dspobslib/Vector Scope  Commented=on  ScopeProperties=on  Domain=User-defined  HorizSpan=1  DisplayProperties=off  AxisGrid=on  Memory=off  FrameNumber=on  AxisLegend=off  AxisZoom=off  OpenScopeAtSimStart=on  OpenScopeImmediately=off  FigPos=get(0,'defaultfigureposition')  AxisProperties=off  XUnits=Hertz  XRange=[0...Fs/2]  InheritXIncr=off  XIncr=1e6/fSraw  XLabel=Time(us)  XLimit=Auto  XMin=0  XMax=1  XStart=0  YUnits=dB  YLabel=Amplitude  LineProperties=off  LineColors=[1 0 0]|[0 1 0]|[0 0 1]  XAxisParamsVer=6.9
      settings: SourceProductName=DSP System Toolbox  SourceProductBaseCode=DS  YMin=-0.6  YMax=0.2
  yTrLramp : dspobslib/Vector Scope  Commented=on  ScopeProperties=on  Domain=User-defined  HorizSpan=1  DisplayProperties=off  AxisGrid=on  Memory=off  FrameNumber=on  AxisLegend=off  AxisZoom=off  OpenScopeAtSimStart=on  OpenScopeImmediately=off  FigPos=get(0,'defaultfigureposition')  AxisProperties=off  XUnits=Hertz  XRange=[0...Fs/2]  InheritXIncr=off  XIncr=1e6/fSraw  XLabel=Time(us)  XLimit=Auto  XMin=0  XMax=1  XStart=0  YUnits=dB  YLabel=Amplitude  LineProperties=off  LineColors=[1 0 0]|[0 1 0]|[0 0 1]  XAxisParamsVer=6.9
      settings: SourceProductName=DSP System Toolbox  SourceProductBaseCode=DS  YMin=-0.6  YMax=0.3
  yTrRamps : dspobslib/Vector Scope  Commented=on  ScopeProperties=on  Domain=User-defined  HorizSpan=1  DisplayProperties=off  AxisGrid=on  Memory=off  FrameNumber=on  AxisLegend=off  AxisZoom=off  OpenScopeAtSimStart=on  OpenScopeImmediately=off  FigPos=get(0,'defaultfigureposition')  AxisProperties=off  XUnits=Hertz  XRange=[0...Fs/2]  InheritXIncr=off  XIncr=1e6/fSdown  XLabel=Time(us)  XLimit=Auto  XMin=0  XMax=1  XStart=0  YUnits=dB  YLabel=Amplitude  LineProperties=off  LineColors=[1 0 0]|[0 1 0]|[0 0 1]  XAxisParamsVer=6.9
      settings: SourceProductName=DSP System Toolbox  SourceProductBaseCode=DS  YMin=-0.6  YMax=0.3
  yTrSync : dspobslib/Vector Scope  Commented=on  ScopeProperties=on  Domain=User-defined  HorizSpan=1  DisplayProperties=off  AxisGrid=on  Memory=off  FrameNumber=on  AxisLegend=off  AxisZoom=off  OpenScopeAtSimStart=on  OpenScopeImmediately=off  FigPos=get(0,'defaultfigureposition')  AxisProperties=off  XUnits=Hertz  XRange=[0...Fs/2]  InheritXIncr=off  XIncr=1e6/fSdown  XLabel=Time(us)  XLimit=Auto  XMin=0  XMax=1  XStart=0  YUnits=dB  YLabel=Amplitude  LineProperties=off  LineColors=[1 0 0]|[0 1 0]|[0 0 1]  XAxisParamsVer=6.9
      settings: SourceProductName=DSP System Toolbox  SourceProductBaseCode=DS  YMin=-0.6  YMax=0.3
  yLoCutOut : Outport
  wires:
  firstTrTime/1(tFtr) -> scaleFactor/2(tFTr), getAntNum/2(tTr), tFramp/1, calcShiftDis/3(tFtr)
  getAntNum/1(iRx) -> iRx/1, calcShiftDis/1(iRx)
  Complex to Real-Imag/1 -> Lowpass Filter/1
  Reshape/1 -> Complex to Real-Imag/1
  interpShiftScale/1(vOut) -> Reshape1/1
  Reshape2/1 -> yLoRamps/1, Assignment/1
  calcTrThres/1(trThres) -> firstTrTime/2(trThres), scaleFactor/3(trThres), Frame Rate Display/1, trThres/1, getAntNum/3(trThres)
  Constant/1 -> Assignment/2
  calcShiftDis/1(dis) -> interpShiftScale1/2(dis), dis/1, interpShiftScale/2(dis)
  Mean/1 -> Reshape2/1
  rawDateIn/1 -> Reshape/1
  Assignment/1 -> yLoCutOut/1, yLoCut/1  "yLoCutSim"
  Reshape4/1 -> yTr/1
  Reshape1/1 -> yLoSync/1, Mean/1
  getAntNum/2(iTx) -> iTx/1, calcShiftDis/2(iTx)
  scaleFactor/2(ysTrLramp) -> Time Scope/1, Array Plot/1, yTrLramp/1
  interpShiftScale1/1(vOut) -> Reshape5/1
  Mean1/1 -> Reshape6/1
  Reshape5/1 -> yTrSync/1, Mean1/1
  Reshape6/1 -> yTrRamps/1
  scaleFactor/1(scFac) -> interpShiftScale1/3(scFac), scFac/1, interpShiftScale/3(scFac)
  Lowpass Filter/1 -> interpShiftScale/1(vIn)
  Complex to Real-Imag/2 -> scaleFactor/1(ysTr), calcTrThres/1(ysTr), firstTrTime/1(ysTr), interpShiftScale1/1(vIn), Reshape4/1, getAntNum/1(ysTr)

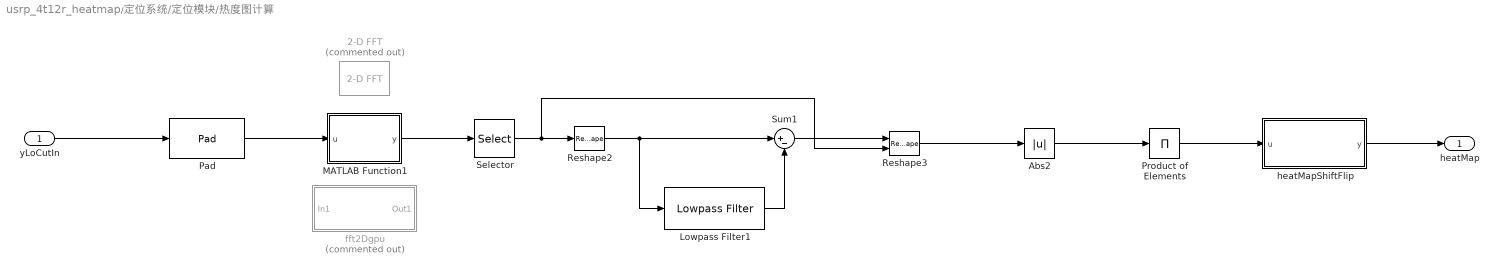
== system usrp_4t12r_heatmap/定位系统/定位模块/热度图计算 ==
  yLoCutIn : Inport
  2-D FFT : visiontransforms/2-D FFT  Commented=on  TableOpt=NEW  TableOptActive=Speed  BitRevOrder=off  SkipNorm=off  FFTImplementation=Auto  firstCoeffDataTypeStr=Inherit: Same word length as input  firstCoeffLastDataTypeStr=Inherit: Same word length as input  outputMin=[]  outputMax=[]  roundingMode=Floor  overflowMode=off
      settings: SourceProductName=Computer Vision System Toolbox  SourceProductBaseCode=VP
  Abs2 : Abs
  Lowpass Filter1 : dspfdesign/Lowpass Filter  FilterType=IIR  DesignForMinimumOrder=off  FilterOrder=1  PassbandFrequency=0.1  StopbandFrequency=3  PassbandRipple=0.1  StopbandAttenuation=30  InheritSampleRate=off  SampleRate=fF  SimulateUsing=Interpreted execution  roundingMode=Floor  coeffsDataTypeStr=fixdt(1,16)
  MATLAB Function1 : MATLAB Function  TreatAsAtomicUnit=on
  Pad : dspsigops/Pad  padAlong=Columns and rows  dimsToPad=1  valSrc=Specify via dialog  padVal=0  spec=Output size  padNumOutRowsSpecMethod=User-specified  numOutRows=lFftDis  padNumOutColsSpecMethod=User-specified  numOutCols=lFftAng  isVarDimsMode=off  padBeginning=0  padEnd=0  outSizeMode=User-specified  outSize=1  padSigAt=End  trunc_flag=None  roundingMode=Floor  overflowMode=off  truncOrWrapMode=Truncate  wrap_flag=None
      settings: SourceProductName=DSP System Toolbox  SourceProductBaseCode=DS
  Product of Elements : Product  Inputs=*  CollapseMode=Specified dimension  CollapseDim=3  OutDataTypeStr=Inherit: Same as first input
  Reshape2 : Reshape  OutputDimensionality=Row vector (2-D)
  Reshape3 : Reshape  OutputDimensionality=Derive from reference input port
  Selector : Selector  NumberOfDimensions=3  InputPortWidth=3  IndexOptions=Index vector (dialog),Select all,Select all  Indices=isDval,1,1  OutputSizes=1,1,1
  Sum1 : Sum  Inputs=|+-
  fft2Dgpu : Subsystem  Commented=on  TreatAsAtomicUnit=on
  heatMapShiftFlip : MATLAB Function  TreatAsAtomicUnit=on
  heatMap : Outport
  wires:
  Pad/1 -> MATLAB Function1/1(u)
  MATLAB Function1/1(y) -> Selector/1
  Lowpass Filter1/1 -> Sum1/2
  Abs2/1 -> Product of Elements/1
  Reshape2/1 -> Lowpass Filter1/1, Sum1/1
  yLoCutIn/1 -> Pad/1
  Product of Elements/1 -> heatMapShiftFlip/1(u)
  Selector/1 -> Reshape3/2, Reshape2/1
  Sum1/1 -> Reshape3/1
  Reshape3/1 -> Abs2/1
  heatMapShiftFlip/1(y) -> heatMap/1

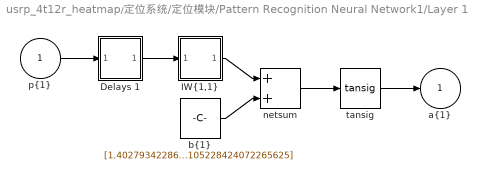
== system usrp_4t12r_heatmap/定位系统/定位模块/Pattern Recognition Neural Network1/Layer 1 ==
  "p{1}" : Inport  PortDimensions=627
      mask Display: e = 0.06;c1 = [120 230 180]/255;c2 = ([120 230 180]+0)/(256+128);c3 = ([120 230 180]+128)/(256+128);patch([0 1 1 0],[0 0 1 1],c1);patch([0 1 1 1-e 1-e 0+e],[0 0 1 1-e 0+e 0+e],c2);patch([0 0 1 1-e 0+e 0+e],[0 1 1 1-e 1-e 0+e],c3);plot([0 1 1 0 0],[0 0 1 1 0]);
  Delays 1 : Subsystem
      mask Display: e = 0.06;c1 = [120 150 230]/255;c2 = ([120 150 230]+0)/383;c3 = ([120 150 230]+128)/383;patch([0 1 1 0],[0 0 1 1],c1);patch([0 1 1 1-e 1-e 0+e],[0 0 1 1-e 0+e 0+e],c2);patch([0 0 1 1-e 0+e 0+e],[0 1 1 1-e 1-e 0+e],c3);plot([0 1 1 0 0],[0 0 1 1 0]);disp('0');
  "IW{1,1}" : Subsystem
      mask Display: e = 0.06;c1 = [120 150 230]/255;c2 = ([120 150 230]+0)/383;c3 = ([120 150 230]+128)/383;patch([0 1 1 0],[0 0 1 1],c1);patch([0 1 1 1-e 1-e 0+e],[0 0 1 1-e 0+e 0+e],c2);patch([0 0 1 1-e 0+e 0+e],[0 1 1 1-e 1-e 0+e],c3);plot([0 1 1 0 0],[0 0 1 1 0]);disp('W');
  "b{1}" : Constant  Value=[1.40279342286191077704415874904952943325042724609375;-1.009089689291936320358900047722272574901580810546875;0.7564906523496663925953953366843052208423614501953125;0.389768104264019588089951184883830137550830841064453125;0.1259307696246152463714906843961216509342193603515625;-0.17571033168955219050388905088766478002071380615234375;-0.40688477505162834457763665341190062463283538818359375;-0.7759938394847811782284452419844456017017364501953125;-1.0394864008526185639169625574140809476375579833984375;1.31738828108706318431586623773910105228424072265625]
      mask Display: e = 0.06;c1 = [120 150 230]/255;c2 = ([120 150 230]+0)/383;c3 = ([120 150 230]+128)/383;patch([0 1 1 0],[0 0 1 1],c1);patch([0 1 1 1-e 1-e 0+e],[0 0 1 1-e 0+e 0+e],c2);patch([0 0 1 1-e 0+e 0+e],[0 1 1 1-e 1-e 0+e],c3);plot([0 1 1 0 0],[0 0 1 1 0]);disp('b');
  netsum : Sum  Inputs=2  SaturateOnIntegerOverflow=on  InputSameDT=on  OutDataTypeStr=Inherit: Same as first input
      mask Display: e = 0.06;c1 = [120 150 230]/255;c2 = ([120 150 230]+0)/383;c3 = ([120 150 230]+128)/383;patch([0 1 1 0],[0 0 1 1],c1);patch([0 1 1 1-e 1-e 0+e],[0 0 1 1-e 0+e 0+e],c2);patch([0 0 1 1-e 0+e 0+e],[0 1 1 1-e 1-e 0+e],c3);plot([0 1 1 0 0],[0 0 1 1 0]);disp('+');
  tansig : neural/Transfer Functions/tansig
  "a{1}" : Outport  InitialOutput=[0;0;0;0;0;0;0;0;0;0]
      mask Display: e = 0.06;c1 = [120 230 180]/255;c2 = ([120 230 180]+0)/(256+128);c3 = ([120 230 180]+128)/(256+128);patch([0 1 1 0],[0 0 1 1],c1);patch([0 1 1 1-e 1-e 0+e],[0 0 1 1-e 0+e 0+e],c2);patch([0 0 1 1-e 0+e 0+e],[0 1 1 1-e 1-e 0+e],c3);plot([0 1 1 0 0],[0 0 1 1 0]);
  wires:
  "p{1}"/1 -> Delays 1/1("p{1}")
  Delays 1/1("pd{1,1}") -> "IW{1,1}"/1("pd{1,1}")
  "IW{1,1}"/1("iz{1,1}") -> netsum/1
  "b{1}"/1 -> netsum/2
  netsum/1 -> tansig/1
  tansig/1 -> "a{1}"/1

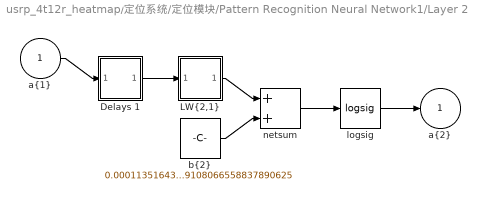
== system usrp_4t12r_heatmap/定位系统/定位模块/Pattern Recognition Neural Network1/Layer 2 ==
  "a{1} " : Inport  PortDimensions=10
      mask Display: e = 0.06;c1 = [120 230 180]/255;c2 = ([120 230 180]+0)/(256+128);c3 = ([120 230 180]+128)/(256+128);patch([0 1 1 0],[0 0 1 1],c1);patch([0 1 1 1-e 1-e 0+e],[0 0 1 1-e 0+e 0+e],c2);patch([0 0 1 1-e 0+e 0+e],[0 1 1 1-e 1-e 0+e],c3);plot([0 1 1 0 0],[0 0 1 1 0]);
  Delays 1 : Subsystem
      mask Display: e = 0.06;c1 = [120 150 230]/255;c2 = ([120 150 230]+0)/383;c3 = ([120 150 230]+128)/383;patch([0 1 1 0],[0 0 1 1],c1);patch([0 1 1 1-e 1-e 0+e],[0 0 1 1-e 0+e 0+e],c2);patch([0 0 1 1-e 0+e 0+e],[0 1 1 1-e 1-e 0+e],c3);plot([0 1 1 0 0],[0 0 1 1 0]);disp('0');
  "LW{2,1}" : Subsystem
      mask Display: e = 0.06;c1 = [120 150 230]/255;c2 = ([120 150 230]+0)/383;c3 = ([120 150 230]+128)/383;patch([0 1 1 0],[0 0 1 1],c1);patch([0 1 1 1-e 1-e 0+e],[0 0 1 1-e 0+e 0+e],c2);patch([0 0 1 1-e 0+e 0+e],[0 1 1 1-e 1-e 0+e],c3);plot([0 1 1 0 0],[0 0 1 1 0]);disp('W');
  "b{2}" : Constant  Value=0.00011351643883979732098377102289532558643259108066558837890625
      mask Display: e = 0.06;c1 = [120 150 230]/255;c2 = ([120 150 230]+0)/383;c3 = ([120 150 230]+128)/383;patch([0 1 1 0],[0 0 1 1],c1);patch([0 1 1 1-e 1-e 0+e],[0 0 1 1-e 0+e 0+e],c2);patch([0 0 1 1-e 0+e 0+e],[0 1 1 1-e 1-e 0+e],c3);plot([0 1 1 0 0],[0 0 1 1 0]);disp('b');
  logsig : neural/Transfer Functions/logsig
      settings: SourceProductName=Neural Network Toolbox  SourceProductBaseCode=NN
  netsum : Sum  Inputs=2  SaturateOnIntegerOverflow=on  InputSameDT=on  OutDataTypeStr=Inherit: Same as first input
      mask Display: e = 0.06;c1 = [120 150 230]/255;c2 = ([120 150 230]+0)/383;c3 = ([120 150 230]+128)/383;patch([0 1 1 0],[0 0 1 1],c1);patch([0 1 1 1-e 1-e 0+e],[0 0 1 1-e 0+e 0+e],c2);patch([0 0 1 1-e 0+e 0+e],[0 1 1 1-e 1-e 0+e],c3);plot([0 1 1 0 0],[0 0 1 1 0]);disp('+');
  "a{2}" : Outport  InitialOutput=0
      mask Display: e = 0.06;c1 = [120 230 180]/255;c2 = ([120 230 180]+0)/(256+128);c3 = ([120 230 180]+128)/(256+128);patch([0 1 1 0],[0 0 1 1],c1);patch([0 1 1 1-e 1-e 0+e],[0 0 1 1-e 0+e 0+e],c2);patch([0 0 1 1-e 0+e 0+e],[0 1 1 1-e 1-e 0+e],c3);plot([0 1 1 0 0],[0 0 1 1 0]);
  wires:
  "a{1} "/1 -> Delays 1/1("p{2}")
  Delays 1/1("pd{2,1}") -> "LW{2,1}"/1("ad{2,1}")
  "LW{2,1}"/1("lz{2,1}") -> netsum/1
  "b{2}"/1 -> netsum/2
  netsum/1 -> logsig/1
  logsig/1 -> "a{2}"/1
